simulink subsystem "Subsystem_Driver_Cruise_BAv02"  (R2022b)
settings: Solver=VariableStepAuto  StartTime=0.0  StopTime=10.0  RelTol=1e-3
settings Model: Creator=giaco  LastModifiedBy=giaco

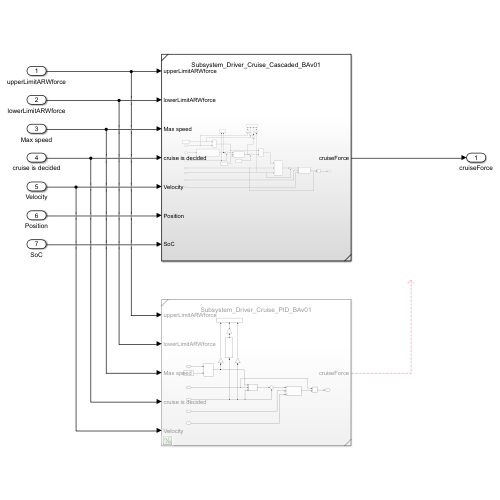
[thumbnail: Simulink's stored preview of the top-level diagram]
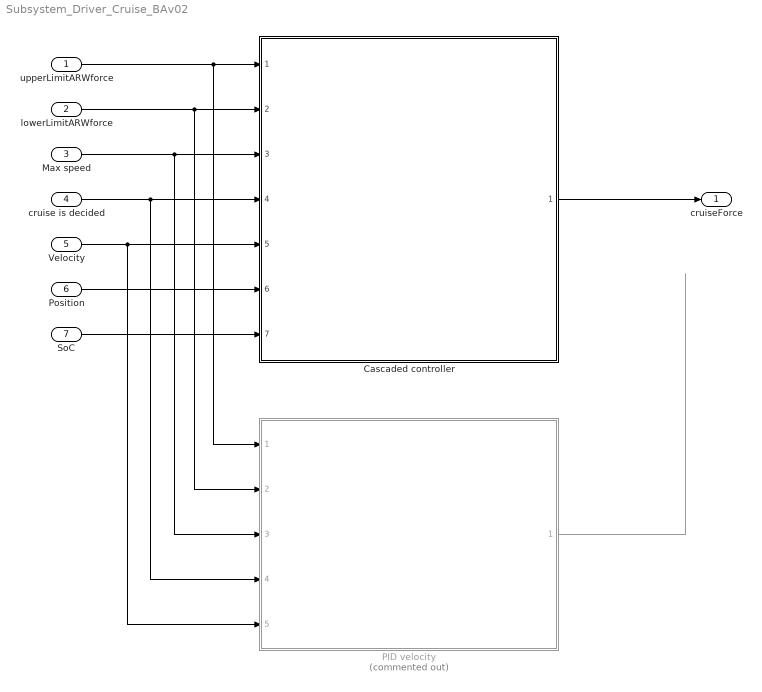
== system Subsystem_Driver_Cruise_BAv02 ==
  upperLimitARWforce : Inport
  lowerLimitARWforce : Inport  Port=2
  Max speed : Inport  Port=3
  cruise is decided : Inport  Port=4
  Velocity : Inport  Port=5
  Position : Inport  Port=6
  SoC : Inport  Port=7
  Cascaded controller : Subsystem  ReferencedSubsystem=Subsystem_Driver_Cruise_Cascaded_BAv02
  PID velocity : Subsystem  Commented=on  ReferencedSubsystem=Subsystem_Driver_Cruise_PID_BAv02
  cruiseForce : Outport
  wires:
  Max speed/1 -> PID velocity/3, Cascaded controller/3
  Position/1 -> Cascaded controller/6
  cruise is decided/1 -> PID velocity/4, Cascaded controller/4
  SoC/1 -> Cascaded controller/7
  Velocity/1 -> PID velocity/5, Cascaded controller/5
  upperLimitARWforce/1 -> PID velocity/1, Cascaded controller/1
  lowerLimitARWforce/1 -> PID velocity/2, Cascaded controller/2
  Cascaded controller/1 -> cruiseForce/1
  PID velocity/1 -> ?
